simulink model "simu"  (R2018b)
settings: Solver=VariableStepAuto  StartTime=0.0  StopTime=30  RelTol=1e-3
values from neighbouring files (symbols this model uses):
  A = [0      1              0           0 ... (first row only)    [intento.m]    (also in prueba.m; task.m = [0,                     0,          0,                      ; task_LQR.m = [             0, 1, 0,                   0; task_PID.m = [             0, 1, 0,                   0)
  B = [     0 ... (first row only)    [intento.m]    (also in prueba.m; task.m = [0; 1/(L*mc); 0; 1/mc]; task_LQR.m = [0; -M*L/p; 0; (I+M*L^2)/p]; task_PID.m = [0; -M*L/p; 0; (I+M*L^2)/p])
  C = [1 0 0 0 ... (first row only)    [intento.m]    (also in prueba.m = [0 0 1 0; 0 0 0 1; 1 0 0 0; 0 1 0 0]; task.m = [1;0;0;0])
  D = [0 ... (first row only)    [intento.m]    (also in prueba.m = zeros(4,1); task.m = 0)
  K = lqr(A,B,Q,R)    [intento.m]    (also in prueba.m = K*C; task.m = [K1; K2; K3; K4]; task_LQR.m = [K_angulo; K_rate; K_pos; K_vel]; task_PID.m = [K_angulo; K_rate; K_pos; K_vel])
  x0 = [0.2; 0; 0; 0]    [intento.m]    (also in prueba.m = [0; 0; 0.2; 0]; task.m = [5*pi/180; 0; 0; 0]; task_LQR.m; task_PID.m)
settings Model: Creator=vuvux  LastModifiedBy=vuvux

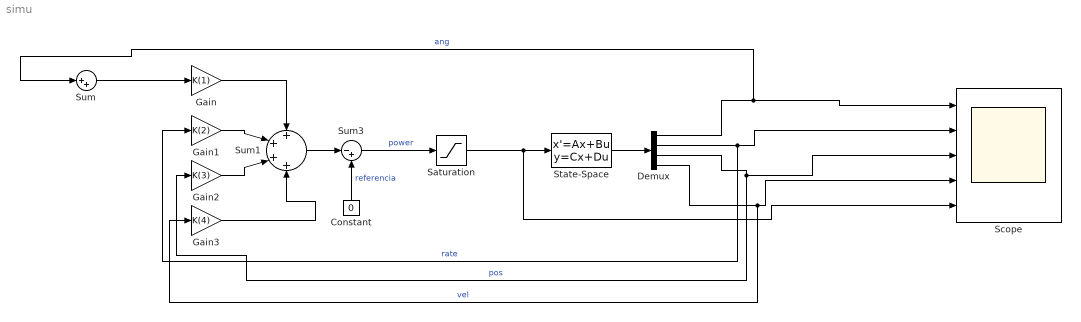
== system simu ==
  Constant : Constant  Value=0
  Demux : Demux
  Gain : Gain  Gain=K(1)
  Gain1 : Gain  Gain=K(2)
  Gain2 : Gain  Gain=K(3)
  Gain3 : Gain  Gain=K(4)
  Saturation : Saturate  UpperLimit=10  LowerLimit=-10
  Scope : Scope  NumInputPorts=5
  State-Space : StateSpace  A=A  B=B  C=C  D=D  InitialCondition=x0
  Sum : Sum  Inputs=|++
  Sum1 : Sum  Inputs=++++
  Sum3 : Sum  Inputs=|-+
  wires:
  State-Space/1 -> Demux/1
  Demux/1 -> Sum/1, Scope/1  "ang"
  Demux/2 -> Gain1/1, Scope/2  "rate"
  Demux/3 -> Scope/3, Gain2/1  "pos"
  Demux/4 -> Scope/4, Gain3/1  "vel"
  Sum/1 -> Gain/1
  Sum1/1 -> Sum3/1
  Constant/1 -> Sum3/2  "referencia"
  Gain/1 -> Sum1/1
  Gain1/1 -> Sum1/2
  Gain2/1 -> Sum1/3
  Gain3/1 -> Sum1/4
  Sum3/1 -> Saturation/1  "power"
  Saturation/1 -> Scope/5, State-Space/1
